simulink model "CANsend"  (R2016b)
settings: Solver=FixedStepDiscrete  StartTime=0.0  StopTime=10.0  FixedStep=1e-3  RelTol=1e-3
libraries: mbed_lib x8
settings Model: Creator=EW  LastModifiedBy=oh
settings DataIOCC: LimitDataPoints=on  SaveFormat=Array
settings OptimizationCC: LifeSpan=1
settings DebuggingCC: SFUnexpectedBacktrackingDiag=warning  SFNoUnconditionalDefaultTransitionDiag=warning  SFExecutionAtInitializationDiag=none
settings HardwareCC: ProdBitPerPointer=32  ProdBitPerSizeT=32  ProdBitPerPtrDiffT=32  ProdLargestAtomicInteger=Long  ProdLargestAtomicFloat=Double  ProdIntDivRoundTo=Undefined  ProdWordSize=32  ProdHWDeviceType=ARM Compatible->ARM Cortex
settings ModelReferenceCC: PropagateSignalLabelsOutOfModel=off
settings RTWCC: SystemTargetFile=mbed.tlc  TemplateMakefile=mbed.tmf  Description=Mbed Target (Embedded Target)  TargetLang=C++
settings CodeAppCC: IgnoreCustomStorageClasses=off
settings STFCustomTargetCC: TargetLibSuffix=.a  GenerateSampleERTMain=on  CombineOutputUpdateFcns=on  ERTCustomFileBanners=on  SupportContinuousTime=off  SupportNonInlinedSFcns=off  RemoveResetFunc=on  MATLABClassNameForMDSCustomization=Simulink.SoftwareTarget.ERTCustomization  GRTInterface=off  SystemTargetFile=mbed.tlc
settings ERTTargetCC: GenerateSampleERTMain=on  ParMdlRefBuildCompliant=off  CompOptLevelCompliant=off  ConcurrentExecutionCompliant=off  ERTFirstTimeCompliant=off  ModelStepFunctionPrototypeControlCompliant=off  CPPClassGenCompliant=off  UseToolchainInfoCompliant=off  ERTCustomFileTemplate=mbed_file_process.tlc  ConvertIfToSwitch=off  SuppressUnreachableDefaultCases=off
settings ConfigComp: CovMetricSettings=dw  CovHtmlReporting=on  CovSaveCumulativeToWorkspaceVar=on  CovSaveSingleToWorkspaceVar=on  CovExternalEMLEnable=off

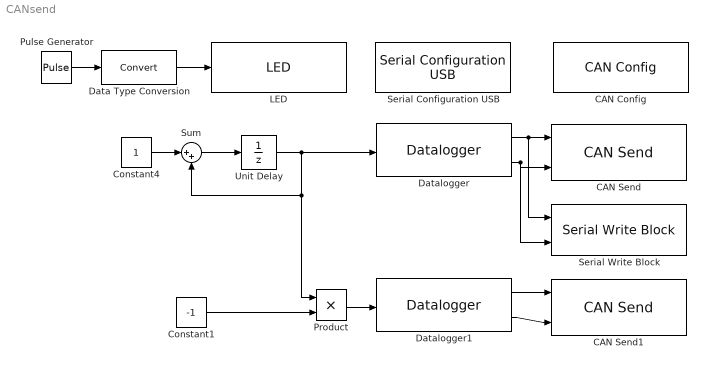
== system CANsend ==
  CAN Config : mbed_lib/Serial/CAN/CAN Config  CAN_ID=1  CAN_frequency=1000000  CAN_Td_Port=A  CAN_Td_Pin=12  CAN_Rd_Port=A  CAN_Rd_Pin=11
  CAN Send : mbed_lib/Serial/CAN/CAN Send  CAN_ID=1  bEnableMsgIDInputport=off  Msg_ID=10  SampleTime=-1
  CAN Send1 : mbed_lib/Serial/CAN/CAN Send  CAN_ID=1  bEnableMsgIDInputport=off  Msg_ID=20  SampleTime=-1
  Constant1 : Constant  Value=-1  OutDataTypeStr=int16  SampleTime=0.5
  Constant4 : Constant  OutDataTypeStr=uint16  SampleTime=1
  Data Type Conversion : DataTypeConversion
  Datalogger : mbed_lib/Utilities/Datalogger  TypeInputPorts={ 'uint16' 1 }  TypeOfInputs={'1*uint16'}  BufferSize=100  errEn=off  SampleTime=-1
  Datalogger1 : mbed_lib/Utilities/Datalogger  TypeInputPorts={ 'int16' 1 }  TypeOfInputs={'1*int16'}  BufferSize=100  errEn=off  SampleTime=-1
  LED : mbed_lib/GPIO/LED  nLED=1  SampleTime=-1
  Product : Product  OutDataTypeStr=int16
  Pulse Generator : DiscretePulseGenerator  PulseType=Time based  Period=1  PulseWidth=50
  Serial Configuration USB : mbed_lib/Serial/UART/Serial Configuration USB  BaudRate=9600
  Serial Write Block : mbed_lib/Serial/UART/Serial Write Block  SerialPort=0  numData=on  SampleTime=-1
  Sum : Sum  Inputs=|++
  Unit Delay : UnitDelay  SampleTime=-1
  wires:
  Unit Delay/1 -> Datalogger/1, Product/1, Sum/2
  Datalogger/2 -> CAN Send/2, Serial Write Block/2
  Datalogger/1 -> CAN Send/1, Serial Write Block/1
  Constant4/1 -> Sum/1
  Sum/1 -> Unit Delay/1
  Datalogger1/1 -> CAN Send1/1
  Datalogger1/2 -> CAN Send1/2
  Product/1 -> Datalogger1/1
  Constant1/1 -> Product/2
  Pulse Generator/1 -> Data Type Conversion/1
  Data Type Conversion/1 -> LED/1
